simulink model "elec_igbt"  (R2014a)
settings: Solver=ode15s  StartTime=0.0  StopTime=t_sim  RelTol=1e-3
PreLoadFcn:
  | Vge = 10;
  | Vce_min = 0;
  | Vce_max = 5;
  | t_sim = 1;
libraries: fl_lib x4, nesl_utility x3, elec_lib x1, simulink x1
Description:
  | IGBT Characteristics
  | 
  | This example shows generation of the Ic versus Vce curve for an
  | insulated gate bipolar transistor. Define the vector of gate-emitter
  | voltages and minimum and maximum collector-emitter voltages by
  | double-clicking the block labeled 'Define Vge and Vce'. Then double
  | click on the block labeled 'Generate Characteristics'.
  | 
  | This type of plot can be compared against a manufacturer
  | datasheet to confirm a correct implementation of the transistor
  | parameters.
  | 
  | 
  | 
  | Copyright 2008-2014 The MathWorks, Inc.
settings Model: FPTRunName=Active  ExtModeAutoUpdateStatusClock=off  Creator=MathWorks  LastModifiedBy=User
settings DataIOCC: SignalLoggingSaveFormat=ModelDataLogs  OutputOption=SpecifiedOutputTimes  OutputTimes=[0:t_sim/100:t_sim]  Refine=5
settings OptimizationCC: ExpressionDepthLimit=2147483647  InitFltsAndDblsToZero=on
settings DebuggingCC: SaveWithParameterizedLinksMsg=none  UnderspecifiedInitializationDetection=Classic  SignalResolutionControl=TryResolveAllWithWarning  SolverPrmCheckMsg=none  FcnCallInpInsideContextMsg=UseLocalSettings  StateNameClashWarn=warning
settings GRTTargetCC: TargetFcnLib=ansi_tfl_tmw.mat  CombineOutputUpdateFcns=off  GRTInterface=on

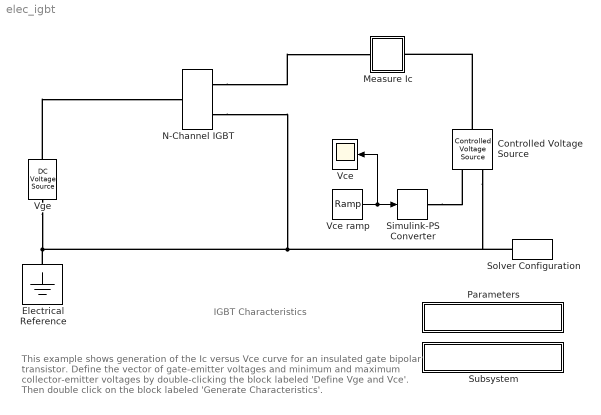
== system elec_igbt ==
  note: IGBT Characteristics
  note: This example shows generation of the Ic versus Vce curve for an insulated
      | gate bipolar transistor. Define the vector of gate-emitter voltages and
      | minimum and maximum collector-emitter voltages by double-clicking the
      | block labeled 'Define Vge and Vce'. Then double click on the block labeled
      | 'Generate Characteristics'.
  Controlled Voltage Source : fl_lib/Electrical/Electrical Sources/Controlled Voltage Source
  Electrical Reference : fl_lib/Electrical/Electrical Elements/Electrical Reference
  Measure Ic : Subsystem
  N-Channel IGBT : elec_lib/Semiconductor Devices/N-Channel IGBT  model_type=1  Ices=2 mA  Vces=600 V  Vth=6 V  Vce_sat=2.6 V  Ice_sat=400 A  Vge_sat=10 V  ec=3  Tmeas=25 C  Vge_vec=[ -2 6 7 8 10 12 15 20 ] V  Vce_vec=[ -1 0 0.5 1 1.5 2 2.5 3 3.5 4 ] V  Ic_mat=[ -1.015e-5 1.35e-8 4.7135e-4 5.092e-4 5.105e-4 5.117500000000001e-4 5.1299e-4 5.1423e-4 5.1548e-4 5.1672e-4; -9.986899999999999e-6 1.35e-8 4.7135e-4 5.092e-4 5.105e-4 5.117500000000001e-4 5.1299e-4 5.1423e-4 5.1548e-4 5.1672e-4; -9.955e-6 1.35e-8 0.0065225 3.3324 48.154 93.661 105.52 105.72 105.93 106.14; -9.955e-6 1.35e-8 0.0065235 3.5783 70.264 166.33 252.4 317.67 353.38 357.39; -9.955e-6 1.35e-8 0.006524 3.7206 89.17100000000001 228.09 371.63 511.02 642.6900000000001 764.04; -9.9549e-6 1.35e-8 0.0065242 3.7716 97.79300000000001 256.21 424.27 592.92 759.2 921.52; -9.9549e-6 1.35e-8 0.0065243 3.8067 104.52 278.11 464.6 654.37 844.5700000000001 1.0339e+3; -9.9549e-6 1.35e-8 0.0065244 3.8324 109.92 295.67 496.54 702.28 909.96 1.1183e+3 ] A  C_param=1  C_GE=23.7 nF  C_GC=2.7 nF  C_ies=26.4 nF  C_res=2.7 nF  C_oes=0 nF  charge_linearity_param=1  C_OX=20 nF  V_C_OX=-5 V  TF=0 us  VAF=200 V  RC=0.001 Ohm  RE=0.001 Ohm  BF=50  T_param=1  Ices_T2=100 mA  EG=1.11 eV  Vce_sat_T2=3 V  Tmeas2=125 C  XTI=3  BEX=-1.5  Tdevice=125 C  Rth=[ 0 10 ] K/W  thermal_mass_parameterization=1  thermal_mass=[ 0 1 ] J/K  thermal_time_constant=[ 0 10 ] s  thermal_mass_initial_temperatures=[ 25 25 ] C
  Parameters : Subsystem  mask(IGBT Test Parameters){Vge_vec=[8 10 12 15 20], Vce_min=0, Vce_max=5, Ic_max=800}
      mask prompts: Vge_vec "Vector of gate-emitter voltages"; Vce_min "Minimum collector-emitter voltage"; Vce_max "Maximum collector-emitter voltage"; Ic_max "Maximum collector current for plotting"
      mask help: Define a range of fixed gate-emitter voltages over which the Ic versus Vce relationship is to be plotted.
      mask Display: disp('Define Vge and Vce')
  Simulink-PS Converter : nesl_utility/Simulink-PS Converter  PhysicalDomain=network_engine_domain  SubClassName=ps_input  LeftPortType=input  RightPortType=output  PseudoPeriodic=off  Frequencies=[]  NoiseDistribution=none  NoiseParameters=[]  Unit=1  AffineConversion=off  InputFiltering=off  SimscapeFilterOrder=1  InputFilterTimeConstant=.001  UdotUserProvided=0
  Solver Configuration : nesl_utility/Solver Configuration  PhysicalDomain=network_engine_domain  SubClassName=solver  LeftPortType=input  RightPortType=generic  Accelerate=off  Tones=[]  Harmonics=[]  SimulateNoise=off  Profile=off  UseLocalSampling=off  EnableSwitchedLinearOptims=on  FrequencyDomain=off  UseCCode=off  RelTol=0.001  AbsTol=1e-06  MinStep=1e-09  ToWorkspace=off  DoDC=on  ResidualTolerance=1e-9  UseLocalSolver=off  LocalSolverChoice=NE_BACKWARD_EULER_ADVANCER  LocalSolverSampleTime=.001  DoFixedCost=off  MaxNonlinIter=3  MaxModeIter=2  LinearAlgebra=Sparse  DelaysMemoryBudget=1024  AutomaticFiltering=on  FilteringTimeConstant=0.001
  Subsystem : Subsystem
      settings: OpenFcn=elec_igbt_callback
      mask Display: disp('Generate Characteristics')
  Vce : Scope
      settings: TimeRange=1  YMin=0  SaveName=Vce
  Vce ramp : simulink/Sources/Ramp  slope=(Vce_max-Vce_min)/t_sim  start=0  X0=Vce_min
  Vge : fl_lib/Electrical/Electrical Sources/DC Voltage Source  v0=Vge V
  wires:
  Vce ramp/1 -> Simulink-PS Converter/1, Vce/1
  connections:
  N-Channel IGBT/RConn2 -- Electrical Reference/LConn1 -- Vge/RConn1 -- Solver Configuration/RConn1 -- Controlled Voltage Source/RConn2
  Vge/LConn1 -- N-Channel IGBT/LConn1
  N-Channel IGBT/RConn1 -- Measure Ic/RConn1
  Controlled Voltage Source/LConn1 -- Measure Ic/LConn1
  Simulink-PS Converter/RConn1 -- Controlled Voltage Source/RConn1

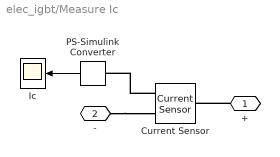
== system elec_igbt/Measure Ic ==
  Current Sensor : fl_lib/Electrical/Electrical Sensors/Current Sensor
  Ic : Scope
      settings: TimeRange=1  YMin=-200  YMax=800  SaveName=Ic
  PS-Simulink Converter : nesl_utility/PS-Simulink Converter  PhysicalDomain=network_engine_domain  SubClassName=ps_output  LeftPortType=input  RightPortType=output  PseudoPeriodic=off  Frequencies=[]  Unit=1  AffineConversion=off
  + : PMIOPort  Port=1  Side=Left
  - : PMIOPort  Port=2  Side=Right
  wires:
  PS-Simulink Converter/1 -> Ic/1
  connections:
  +/RConn1 -- Current Sensor/LConn1
  -/RConn1 -- Current Sensor/RConn2
  Current Sensor/RConn1 -- PS-Simulink Converter/LConn1

== system elec_igbt/Parameters ==

== system elec_igbt/Subsystem ==
